simulink model "bicycle"  (R2017a)
settings: Solver=VariableStepAuto  StartTime=0.0  StopTime=tmax  MaxStep=dt  RelTol=1e-3
StartFcn:
  | clc; clearvars
  | close all
  | %% System Parameters (nominal)
  | % i.e., for this investigation, ...the knobs
  | m = 1452; % Mass of Vehicle (kg)
  | J = 2200; % Moment of Inertia (kg-m^2)
  | Jx = 510; % Roll Moment of Inertia (kg-m^2)
  | L = 2.7; % Wheel base of Vehicle (m)
  | a = 1.120; % Length of a (m)
  | b = L - a; % Length of b (m)
  | h = 0.562; % C.G Height (m)
  | Cf = 50000; % Conering Coefficient of Front Tire (N/rad)
  | Cr = 40000; % Base cornering coefficient
  | Crr = 0.161; % Roll Steer Coefficient of Rear (rad/rad): tune parameter_1
  | ktau = (1006 + 736)*180/pi; % Vehicle Roll Stiffness (Nm/deg*180/pi --> Nm/rad): tune parameter_2
  | Cls = -0.113*pi/180/1000; % Lateral Steer Coefficient of Rear (deg/kN*(pi/180/1000)-->rad/N) : tune parameter_3
  | vx = 28; % Longitudinal Velocity (m/s)== 100kph
  | K = 1; %Understeer Gradient Coefficient
  | %% Time parameters
  | % No need to change
  | tmax = 10;
  | dt = 0.001;
  | %% Initial conditions
  | init = zeros(7,1);
  | p = [m; J; Jx; a; b; h; Cf; Cr; Crr; ktau; Cls; vx];
StopFcn:
  | dx = datasave.get('dx').Values.Data;
  | x = datasave.get('x').Values.Data;
  | z = datasave.get('z').Values.Data;
  | t = datasave.get('t').Values.Data;
  | % Unpack states
  | v = x(:,1);
  | w = x(:,2);
  | psi = x(:,3);
  | X = x(:,4);
  | Y = x(:,5);
  | wx = x(:,6);
  | theta = x(:,7);
  | % Unpack additional outputs
  | ay = z(:,1);
  | del_l2 = z(:,2);
  | del_r2 = z(:,3);
  | beta_b = z(:,4);
  | alf2 = z (:,5);
  | 
  | mets
  | plots
undefined symbols (not defined in the file): sigbuilder_block
settings Model: Creator=zac  LastModifiedBy=zac
settings DataIOCC: SaveFormat=Array  SaveOutput=off  DSMLogging=off  SaveTime=off  SignalLoggingName=datasave

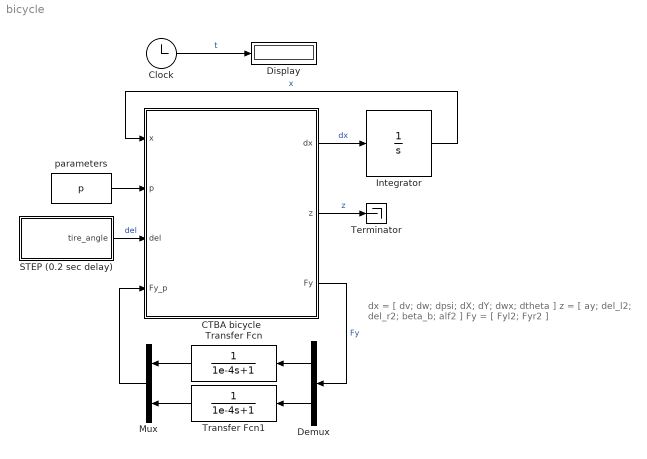
== system bicycle ==
  note: dx = [ dv; dw; dpsi; dX; dY; dwx; dtheta ]
      | z = [ ay; del_l2; del_r2; beta_b; alf2 ]
      | Fy = [ Fyl2; Fyr2 ]
  CTBA bicycle : MATLAB Function  TreatAsAtomicUnit=on
  Clock : Clock
  Demux : Demux  Outputs=2
  Display : Display
  Integrator : Integrator  InitialCondition=init
  Mux : Mux  Inputs=2
  STEP (0.2 sec delay) : Subsystem  Tag=STV Subsys  LoadFcn=sigbuilder_block('load');  StartFcn=sigbuilder_block('start');  StopFcn=sigbuilder_block('stop');  ClipboardFcn=sigbuilder_block('clipboard');  mask(Sigbuilder block){tuvar=[0:10]}
      mask help: Simulink:masks:SigbuilderBlock_MD
      mask init:
      | if ~strcmp(get_param(bdroot(gcbh),'SimulationStatus'),'stopped') tuvar = sigbuilder_block('maskInit'); end
      settings: CopyFcn=sigbuilder_block('copy');  DeleteFcn=sigbuilder_block('delete');  ModelCloseFcn=sigbuilder_block('modelClose');  PreSaveFcn=sigbuilder_block('preSave');  PauseFcn=sigbuilder_block('pause');  ContinueFcn=sigbuilder_block('continue');  NameChangeFcn=sigbuilder_block('namechange');  OpenFcn=sigbuilder_block('open',[567 140.25 550.5 399.75 ]);  CloseFcn=sigbuilder_block('close');
      mask Display: plot(0, 0, 100, 100,[2, 2, 32, 32, 2], [68, 8, 8, 68, 68],[32, 2], [38, 38], [32, 19, 2],[53, 60, 44], [32, 17, 17, 2],[16, 16, 31, 31]);txt = getActiveGroup(gcbh);text(2, 100, txt,'verticalAlignment', 'top');
  Terminator : Terminator
  Transfer Fcn : TransferFcn  Denominator=[1e-4 1]
  Transfer Fcn1 : TransferFcn  Denominator=[1e-4 1]
  parameters : Constant  Value=p
  wires:
  Transfer Fcn1/1 -> Mux/2
  Transfer Fcn/1 -> Mux/1
  Demux/1 -> Transfer Fcn/1
  Demux/2 -> Transfer Fcn1/1
  CTBA bicycle/1(dx) -> Integrator/1  "dx"
  Integrator/1 -> CTBA bicycle/1(x)  "x"
  STEP (0.2 sec delay)/1(tire_angle) -> CTBA bicycle/3(del)  "del"
  CTBA bicycle/3(Fy) -> Demux/1  "Fy"
  Mux/1 -> CTBA bicycle/4(Fy_p)
  CTBA bicycle/2(z) -> Terminator/1  "z"
  Clock/1 -> Display/1  "t"
  parameters/1 -> CTBA bicycle/2(p)

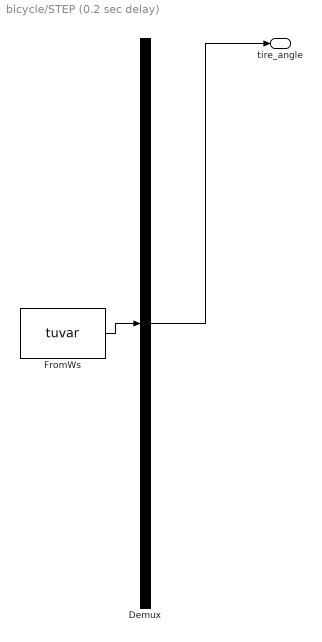
== system bicycle/STEP (0.2 sec delay) ==
  Demux : Demux  Tag=STV Demux  Outputs=1
  FromWs : FromWorkspace  Tag=STV FromWs  VariableName=tuvar  SampleTime=0
      SigBuilderData=|
      | common.afterFinalStr = 'Extrapolate'
      | common.sampleTime = 0
      | dataSet.timeRange = [0 10]
      | dataSet.name = 'steering'
      | sbobj.Groups.Name = 'steering'
      | sbobj.Groups.Signals.Name = 'tire_angle'
      | sbobj.Groups.Signals.XData = [0 2 2.2 10]
      | sbobj.Groups.Signals.YData = [0 0 0.0349065850399 0.0349065850399]
  tire_angle : Outport  Tag=STV Outport
  wires:
  Demux/1 -> tire_angle/1
  FromWs/1 -> Demux/1

== matlab function bicycle/CTBA bicycle ==
  data: x input; p input; dx output; del input; Fy_p input; z output; Fy output
function [dx,z,Fy] = ctbabike(x, p, del, Fy_p)

% m, J, Jx, a, b, h, Cf, Cr, Crr, ktau, Cls, vx

% Unpack states
v = x(1);
w = x(2);
psi = x(3);
% X = x(4);
% Y = x(5);
wx = x(6);
theta = x(7);
% Unpack parameters
m = p(1); J = p(2); Jx = p(3);
a = p(4); b = p(5); h = p(6);
Cf = p(7); Cr = p(8); Crr = p(9);
ktau = p(10); Cls = p(11); vx = p(12);
% Unpack previous tire forces
Fyl2_p = Fy_p(1);
Fyr2_p = Fy_p(2);

% Rear Steer Angle using the previous tire force
del_l2 = Crr*theta + Cls*(Fyl2_p+Fyr2_p); % Rear-left steer angle
del_r2 = Crr*theta + Cls*(Fyl2_p+Fyr2_p); % Rear-right steer angle

% Front and rear slip angles
alf1 = del - (v + a*w)/vx;
alf2 = -(v - b*w)/vx;

% % Equivalent rear axle slip angle
% D = (2*Cr*Crr*h - ktau + 2*Cls*Cr*ktau);
% beta1 = -2*Cf*Crr*h/D;
% beta2 = -ktau/D;
% alf2_mod = beta1*alf1 + beta2*alf2;

% Front tire forces
% - Assume no suspension effects
Fyl1 = Cf*alf1;
Fyr1 = Cf*alf1;

% Rear lateral tire forces
% Fyl2 = Cr*alf2_mod;
% Fyr2 = Cr*alf2_mod;
Fyl2 = Cr*(alf2 + del_l2);
Fyr2 = Cr*(alf2 + del_r2);

% Total lateral tire force
Fy_all = Fyl1 + Fyr1 + Fyl2 + Fyr2;

% Equations of motion
dv = 1/m*Fy_all - w*vx;
dw = 1/J*(a*(Fyl1 + Fyr1) - b*(Fyl2 + Fyr2));
dpsi = w;
dX = vx*cos(psi) - v*sin(psi);
dY = vx*sin(psi) + v*cos(psi);
dwx = 1/Jx*(-ktau*theta + Fy_all*h - 4*(1.5/2)^2*2.9400e+03*wx); %-4*(1.5/2)^2*2.9400e+03*wx
dtheta = wx;

% Additional outputs
ay = dv + vx*w; % Lateral acceleration
% del_l2 = Crr*Fy_all*h/ktau + Cls*(Fyl2 + Fyr2); % Rear-left steer angle
% del_r2 = Crr*Fy_all*h/ktau + Cls*(Fyl2 + Fyr2); % Rear-right steer angle
beta_b = atan(v/vx); % Body slip angle

% Pack output vectors
dx = [dv; dw; dpsi; dX; dY; dwx; dtheta];
z = [ay; del_l2; del_r2; beta_b; alf2];
Fy = [Fyl2;Fyr2];
